simulink model "Temporal3"  (R2020a)
settings: Solver=VariableStepAuto  StartTime=0.0  StopTime=1.0  RelTol=1e-3
settings Model: Creator=86188  LastModifiedBy=bzhan
settings DataIOCC: ReturnWorkspaceOutputs=off
settings DebuggingCC: ArithmeticOperatorsInVariantConditions=warning
settings SFSimCC: SimUseLocalCustomCode=off  CustomCodeUndefinedFunction=UseInterfaceOnly
settings RTWCC: RTWUseLocalCustomCode=off

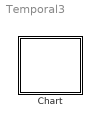
== system Temporal3 ==
  Chart : Stateflow chart  TreatAsAtomicUnit=on

== stateflow chart Temporal3/Chart ==
  settings: updateMethod=DISCRETE  sampleTime=0.1
  state A
    en:f("en_A");
    x=1;
    du:f("du_A");
    x=x+1;
  state B
    en:f("en_B")
    du:f("du_B");
  (default) -> A
  A -> B : after(3,tick)[x>=5]
  B -> A : after(3,tick)
  data: s function_input; x local
  function f(s):
    | function f(s)
    |   fprintf(s+"\n");
